simulink model "JX_Kinect_multi_sync"  (Simulink 7.7)
settings: Solver=ode4  StartTime=0.0  StopTime=inf  FixedStep=sample_time  RelTol=1e-3
InitFcn:
  | sample_time=0.005;%0.004;%0.0025;%0.02;
  | DeltaT = 0.02;
  | g = 9.81;
  | H0 = g%0.3165;
  | Kl = 1;
  | 
  | Omega_r = 1.6;%for Horizontal reference
  | Zeta_r = 1; %for Horizontal reference
  | Omega = 1.8;%for Horizontal Control
  | Zeta = 0.5;    %for Horizontal Control
  | 
  | Omega_h_r = 2.5; %for vertical reference
  | Zeta_h_r = 0.8;  %for vertical reference
  | Omega_h = 2.7;    %for vertical control
  | Zeta_h = 0.8;         %for vertical control
  | PI=pi;
  | 
  | Mass = 1.15;
  | Acc_Max = 4;
  | Acc_Max_h = 4;
  | 
  | Max_RP = 60;
  | 
  | % for NN
  | n = 5;
  | r = 3;
  | n2 = 5;
  | NN_ST = 0.02;
  | 
  | GAMA_V = 6;
  | gama_V_e = 0.01;
  | 
  | GAMA_W = GAMA_V;
  | gama_W_e =0.01;
  | 
  | % deadzone
  | NN_Deadzone_Z = 0;
  | 
  | % inputs nomalizaton parameters
  | NN_Z_y_min = -3;
  | NN_Z_y_max = 0.5;
  | 
  | NN_Z_v_max = 8;
  | NN_Z_v_min = -NN_Z_v_max;
  | 
  | % alpha = 0.034;
  | alpha = 1;
  | % c_f = 0.0015;
  | c_f = 0.001;
  | c_y_tilt = 1*0.5;
  | 
  | %for WK paras
  | Heightcontrol = 0.08;
  | Scale_Factor=1;
  | yoffset=0;
  | 
  | load MaoBi_Oct04_2_int.mat
  | MB_Interp.time = [];
undefined symbols (not defined in the file or in its folder): DiscIntNeverNeededParam
libraries: simulink x15, X330_Control x6, dspadpt3 x6, nid_lib x2
(part 4 of 4)

== system JX_Kinect_multi_sync/Vicon_Data/Raw Quad Pose from Vicon/Process Vicon Raw Data2/Flip_pi1/Flip_0_to_2pi/Flip_2pi ==
  Angle : Inport
  Bias : Bias  Bias=-2*pi
  Constant : Constant  Value=2*pi
  Data Type Duplicate : DataTypeDuplicate
  Modulo : Math  Operator=mod  SaturateOnIntegerOverflow=on
  Sign1 : Signum
  Switch : Switch
  Angle_Flip : Outport
  wires:
  Switch/1 -> Data Type Duplicate/2, Angle_Flip/1
  Bias/1 -> Switch/3
  Sign1/1 -> Switch/2
  Modulo/1 -> Switch/1, Bias/1
  Constant/1 -> Modulo/2
  Angle/1 -> Data Type Duplicate/1, Sign1/1, Modulo/1

== system JX_Kinect_multi_sync/Vicon_Data/Raw Quad Pose from Vicon/Process Vicon Raw Data3/Flip_pi1/Flip_0_to_2pi/Flip_2pi ==
  Angle : Inport
  Bias : Bias  Bias=-2*pi
  Constant : Constant  Value=2*pi
  Data Type Duplicate : DataTypeDuplicate
  Modulo : Math  Operator=mod  SaturateOnIntegerOverflow=on
  Sign1 : Signum
  Switch : Switch
  Angle_Flip : Outport
  wires:
  Angle/1 -> Modulo/1, Sign1/1, Data Type Duplicate/1
  Constant/1 -> Modulo/2
  Modulo/1 -> Bias/1, Switch/1
  Sign1/1 -> Switch/2
  Bias/1 -> Switch/3
  Switch/1 -> Angle_Flip/1, Data Type Duplicate/2

== system JX_Kinect_multi_sync/Vicon_Data/Raw Quad Pose from Vicon/Process Vicon Raw Data4/Flip_pi1/Flip_0_to_2pi/Flip_2pi ==
  Angle : Inport
  Bias : Bias  Bias=-2*pi
  Constant : Constant  Value=2*pi
  Data Type Duplicate : DataTypeDuplicate
  Modulo : Math  Operator=mod  SaturateOnIntegerOverflow=on
  Sign1 : Signum
  Switch : Switch
  Angle_Flip : Outport
  wires:
  Switch/1 -> Data Type Duplicate/2, Angle_Flip/1
  Bias/1 -> Switch/3
  Sign1/1 -> Switch/2
  Modulo/1 -> Switch/1, Bias/1
  Constant/1 -> Modulo/2
  Angle/1 -> Data Type Duplicate/1, Sign1/1, Modulo/1

== system JX_Kinect_multi_sync/Vicon_Data/Raw Quad Pose from Vicon/Process Vicon Raw Data6/Flip_pi1/Flip_0_to_2pi/Flip_2pi ==
  Angle : Inport
  Bias : Bias  Bias=-2*pi
  Constant : Constant  Value=2*pi
  Data Type Duplicate : DataTypeDuplicate
  Modulo : Math  Operator=mod  SaturateOnIntegerOverflow=on
  Sign1 : Signum
  Switch : Switch
  Angle_Flip : Outport
  wires:
  Angle/1 -> Modulo/1, Sign1/1, Data Type Duplicate/1
  Constant/1 -> Modulo/2
  Modulo/1 -> Bias/1, Switch/1
  Sign1/1 -> Switch/2
  Bias/1 -> Switch/3
  Switch/1 -> Angle_Flip/1, Data Type Duplicate/2

== system JX_Kinect_multi_sync/Vicon_Data/Raw Quad Pose from Vicon/Process Vicon Raw Data7/Flip_pi1/Flip_0_to_2pi/Flip_2pi ==
  Angle : Inport
  Bias : Bias  Bias=-2*pi
  Constant : Constant  Value=2*pi
  Data Type Duplicate : DataTypeDuplicate
  Modulo : Math  Operator=mod  SaturateOnIntegerOverflow=on
  Sign1 : Signum
  Switch : Switch
  Angle_Flip : Outport
  wires:
  Switch/1 -> Data Type Duplicate/2, Angle_Flip/1
  Bias/1 -> Switch/3
  Sign1/1 -> Switch/2
  Modulo/1 -> Switch/1, Bias/1
  Constant/1 -> Modulo/2
  Angle/1 -> Data Type Duplicate/1, Sign1/1, Modulo/1

== matlab function UAV1/Yaw Controller/MATLAB Function ==
  data: u input double; y output double
function y = fcn(u)
%#codegen
y = u;
if y > pi    
    y = y - 2*pi;
elseif y < -pi
        y = y + 2*pi;
end

== stateflow chart UAV2/Trajectory Logic/UAV SF ==
  state Landing
    state Descending
      en:PosDesired = Pos;
      du:PosDesired[2] = (0.1- PosDesired[2])*1*DeltaT + PosDesired[2] ;
    state CutThrottle
      en: PWM=1600;
      du:HoverThrottle = (0.0- HoverThrottle)*3*DeltaT + HoverThrottle ;
    (default) -> Descending
    Descending -> CutThrottle : [Pos[2] >(0.0 -0.1)]
  state AirBorne
    state TakeOff
      du:HoverThrottle = (H0 - HoverThrottle)*3*DeltaT + HoverThrottle ;
    state Kinect
      state Initialise
        en:
        PosDesired[0]=-1.5, PosDesired[1]=0,PosDesired[2]= -1.5,PosDesired[3]=0;
        LeftRight = 0;
        UpDown = 0;
        FrontBack = 0;
      state UpdateQuad
        en:
        PosDesired[0]=LeftRight, PosDesired[1]=FrontBack,PosDesired[2]=UpDown;
      state Kinect
        state FollowKinect
          en:
          LeftRight = KPos[3], FrontBack = KPos[4], UpDown = KPos[5];
          LH=1;
        state BoundaryContact
          en:
          LH=1;
        (default) -> (junction 41)
        (junction 41) -> BoundaryContact [order 2] : [((TooClose[0]==1)&(TooClose[2]==0))|((TooClose[0]==0)&(TooClose[2]==1))|(TooClose[3]==1)]
        (junction 41) -> FollowKinect [order 1] : [(TooClose[0]==0)&(TooClose[2]==0)]
      state Constraint
        state ALLGreen
          en:
          LH = 2;
        state PositionConstraint
          state Znegative
            en:
            UpDown=-2.5;
          state Ynegative
            en:
            FrontBack=-2;
          state Zpositive
            en:
            UpDown=-0.8;
          state Contained
            en:
            LH = 2;
          state Xpositive
            en:
            LeftRight=2;
          state Xnegative
            en:
            LeftRight=-2;
          state Ypositive
            en:
            FrontBack=2;
          Znegative -> Contained
          (junction 39) -> Zpositive [order 2] : [UpDown>-0.8]
          (junction 40) -> (junction 39) [order 1] : [FrontBack>=-2]
          Zpositive -> (junction 38)
          (junction 38) -> Znegative [order 2] : [UpDown<-2.5]
          (junction 39) -> (junction 38) [order 1] : [UpDown<=-0.8]
          (junction 38) -> Contained [order 1] : [UpDown>=-2.5]
          Ynegative -> (junction 39)
          (default) -> (junction 43)
          (junction 43) -> Xpositive [order 2] : [LeftRight>2]
          (junction 43) -> (junction 37) [order 1] : [LeftRight<=2]
          Xpositive -> (junction 37)
          (junction 37) -> Xnegative [order 2] : [LeftRight<-2]
          Xnegative -> (junction 36)
          (junction 37) -> (junction 36) [order 1] : [LeftRight>=-2]
          (junction 36) -> Ypositive [order 2] : [FrontBack>2]
          Ypositive -> (junction 40)
          (junction 36) -> (junction 40) [order 1] : [FrontBack<=2]
          (junction 40) -> Ynegative [order 2] : [FrontBack<-2]
        (default) -> (junction 42)
        (junction 42) -> ALLGreen [order 1] : [(LeftRight<=2)&(LeftRight>=-2)&(FrontBack<=2)&(FrontBack>=-2)&(UpDown<=-0.8)&(UpDown>=-2.5)]
        (junction 42) -> PositionConstraint [order 2] : [(LeftRight > 2)|(LeftRight<-2)|(FrontBack>2)|(FrontBack<-2)|(UpDown>-0.8)|(UpDown<-2.5)]
        PositionConstraint -> ALLGreen : [(LeftRight<=2)&(LeftRight>=-2)&(FrontBack<=2)&(FrontBack>=-2)&(UpDown<=-0.8)&(UpDown>=-2.5)]
      (default) -> Initialise
      Initialise -> UpdateQuad : after (3,sec)
      AirBorne.Kinect.Kinect -> UpdateQuad [order 1] : [KinectTracking==0]
      UpdateQuad -> AirBorne.Kinect.Kinect : [KinectTracking==1]
      Constraint -> UpdateQuad : [LH==2]
      AirBorne.Kinect.Kinect -> Constraint [order 2] : [LH==1]
    state Safety
      state Descent1
        descentrate=descentrate+0.02;
      state Prelanding
        en:PosDesired[0] = PerchPos[0]; PosDesired[1] = PerchPos[1];PosDesired[2] = PerchPos[2]-0.8 ;
        descentrate=0;
      state SafyHover
        en:PosDesired = Pos; PosDesired[2]= -1.5;
      state Descent
        en:PosDesired[0] = PerchPos[0]; PosDesired[1] = PerchPos[1];PosDesired[2] = PerchPos[2]-0.50+descentrate;
      Prelanding -> Descent : [PerchError < 0.01]
      Descent -> Descent1 [order 2] : [PerchError < 0.02]
      (default) -> SafyHover
      Descent -> Prelanding [order 1] : after (5,sec)
      Descent1 -> Descent : after (0.5,sec)
      SafyHover -> Prelanding : after (3, sec)
    (default) -> TakeOff : {PosDesired = Pos;  PosDesired[2] =-1.2;}
    TakeOff -> Safety [order 2] : [RC[5] > 0.5]
    TakeOff -> AirBorne.Kinect [order 1] : after (7,sec)
    AirBorne.Kinect -> Safety : [RC[5] > 0.5]
  (default) -> Landing : {HoverThrottle = 0;}
  AirBorne -> Landing : [RC[6] < -0.5]
  Landing -> AirBorne : [RC[6] > 0.5]
  data: PosDesired output double size=4; HoverThrottle output double size=1; Mode output uint8 size=1; RC input double size=8; Pos input double size=4; PerchPos input double size=4; DeltaT parameter double size=1; H0 parameter double size=1; Kl parameter double size=1; VelCmd local double size=2 =0; PWM output double; PerchError input double; KinectTracking input double; PI parameter double size=1; descentrate local double; KPos input double; UpDown local double; FrontBack local double; TooClose input double; LeftRight local double; XDiff local double; YDiff local double; diff local double; LH local double

== stateflow chart UAV1/Trajectory Logic/UAV SF ==
  state Landing
    state Descending
      en:PosDesired = Pos;
      du:PosDesired[2] = (0.1- PosDesired[2])*1*DeltaT + PosDesired[2] ;
    state CutThrottle
      en: PWM=1600;
      du:HoverThrottle = (0.0- HoverThrottle)*3*DeltaT + HoverThrottle ;
    (default) -> Descending
    Descending -> CutThrottle : [Pos[2] >(0.0 -0.1)]
  state AirBorne
    state TakeOff
      du:HoverThrottle = (H0 - HoverThrottle)*3*DeltaT + HoverThrottle ;
    state Kinect
      state Initialise
        en:
        PosDesired[0]=-1.5, PosDesired[1]=0,PosDesired[2]= -1.5,PosDesired[3]=0;
        LeftRight = 0;
        UpDown = 0;
        FrontBack = 0;
      state UpdateQuad
        en:
        PosDesired[0]=Pos2[0]+LeftRight, PosDesired[1]=Pos2[1]+FrontBack,PosDesired[2]= Pos2[2]+UpDown;
      state Kinect
        state FollowKinect
          en:
          LeftRight = KPos[0], FrontBack = KPos[1], UpDown = KPos[2];
          LH=1;
        state AtLeast2BoundaryContact
          state xright
            en:
            LeftRight = LeftRight+0.05;
            LH=1;
          state xleft
            en:
            LeftRight = LeftRight-0.05;
            LH=1;
          state yfront
            en:
            FrontBack = FrontBack-0.05;
            LH=1;
          state xright1
            en:
            FrontBack = FrontBack+0.05;
            LH=1;
          state quad3
            en:
            LH=1;
          (default) -> (junction 149)
          (junction 149) -> (junction 150) [order 2] : [TooClose[4]>TooClose[5]]
          (junction 149) -> (junction 151) [order 1] : [TooClose[5]>=TooClose[4]]
          (junction 150) -> (junction 152) [order 2] : [TooClose[6]==1]
          (junction 151) -> (junction 153) [order 1] : [TooClose[7]==1]
          (junction 152) -> xleft [order 2] : [KPos[0]<0]
          (junction 152) -> xright [order 1] : [KPos[0]>=0]
          (junction 153) -> yfront [order 2] : [KPos[1]<0]
          (junction 153) -> xright1 [order 1] : [KPos[1]>=0]
          (junction 150) -> quad3 [order 1] : [TooClose[6]==0]
          (junction 151) -> quad3 [order 2] : [TooClose[7]==0]
        state OneBoundaryContact
          en:
          LH=1;
        (default) -> (junction 154)
        (junction 154) -> AtLeast2BoundaryContact [order 2] : [TooClose[3]==1]
        (junction 154) -> FollowKinect [order 3] : [(TooClose[0]==0)&(TooClose[1]==0)]
        (junction 154) -> OneBoundaryContact [order 1] : [((TooClose[0]==1)&(TooClose[1]==0))|((TooClose[0]==10)&(TooClose[1]==1))]
      state Constraint
        state ALLGreen
          en:
          LH = 2;
        state PositionConstraint
          state Xpositive
            en:
            LeftRight=(2-Pos2[0]);
          state Xnegative
            en:
            LeftRight=(-2-Pos2[0]);
          state Ypositive
            en:
            FrontBack=(2-Pos2[1]);
          state Ynegative
            en:
            FrontBack=(-2-Pos2[1]);
          state Zpositive
            en:
            UpDown=(0.78-Pos2[2]);
          state Znegative
            en:
            UpDown=(-1-Pos2[2]);
          state Contained
            en:
            LH = 2;
          (default) -> (junction 156)
          (junction 156) -> Xpositive [order 2] : [LeftRight>(2-Pos2[0])]
          (junction 156) -> (junction 157) [order 1] : [LeftRight<=(2-Pos2[0])]
          Xpositive -> (junction 157)
          (junction 157) -> Xnegative [order 2] : [LeftRight<(-2-Pos2[0])]
          Xnegative -> (junction 158)
          (junction 157) -> (junction 158) [order 1] : [LeftRight>=(-2-Pos2[0])]
          (junction 158) -> Ypositive [order 2] : [FrontBack>(2-Pos2[1])]
          Ypositive -> (junction 159)
          (junction 158) -> (junction 159) [order 1] : [FrontBack<=(2-Pos2[1])]
          (junction 159) -> Ynegative [order 2] : [FrontBack<(-2-Pos2[1])]
          Ynegative -> (junction 160)
          (junction 159) -> (junction 160) [order 1] : [FrontBack>=(-2-Pos2[1])]
          (junction 160) -> Zpositive [order 2] : [UpDown>(0.78-Pos2[2])]
          Zpositive -> (junction 161)
          (junction 160) -> (junction 161) [order 1] : [UpDown<=(0.78-Pos2[2])]
          (junction 161) -> Znegative [order 2] : [UpDown<(-1-Pos2[2])]
          (junction 161) -> Contained [order 1] : [UpDown>=(-1-Pos2[2])]
          Znegative -> Contained
        (default) -> (junction 155)
        (junction 155) -> ALLGreen [order 1] : [(LeftRight<=(2-Pos2[0]))&(LeftRight>=(-2-Pos2[0]))&(FrontBack<=(2-Pos2[1]))&(FrontBack>=(-2-Pos2[1]))&(UpDown<=(0.78-Pos2[2]))&(UpDown>=(-1-Pos2[2]))]
        (junction 155) -> PositionConstraint [order 2] : [(LeftRight > (2-Pos2[0]))|(LeftRight<(-2-Pos2[0]))|(FrontBack>(2-Pos2[1]))|(FrontBack<(-2-Pos2[1]))|(UpDown>(0.78-Pos2[2]))|(UpDown<(-1-Pos2[2]))]
        PositionConstraint -> ALLGreen : [(LeftRight<=(2-Pos2[0]))&(LeftRight>=(-2-Pos2[0]))&(FrontBack<=(2-Pos2[1]))&(FrontBack>=(-2-Pos2[1]))&(UpDown<=(0.78-Pos2[2]))&(UpDown>=(-1-Pos2[2]))]
      (default) -> Initialise
      Initialise -> UpdateQuad : after (3,sec)
      AirBorne.Kinect.Kinect -> UpdateQuad [order 1] : [KinectTracking==0]
      UpdateQuad -> AirBorne.Kinect.Kinect : [KinectTracking==1]
      AirBorne.Kinect.Kinect -> Constraint [order 2] : [LH==1]
      Constraint -> UpdateQuad : [LH==2]
    state Safety
      state Descent1
        descentrate=descentrate+0.02;
      state Prelanding
        en:PosDesired[0] = PerchPos[0]; PosDesired[1] = PerchPos[1];PosDesired[2] = PerchPos[2]-0.8 ;
        descentrate=0;
      state SafyHover
        en:PosDesired = Pos; PosDesired[2]= -1.5;
      state Descent
        en:PosDesired[0] = PerchPos[0]; PosDesired[1] = PerchPos[1];PosDesired[2] = PerchPos[2]-0.50+descentrate;
      Prelanding -> Descent : [PerchError < 0.01]
      Descent -> Descent1 [order 2] : [PerchError < 0.02]
      (default) -> SafyHover
      Descent -> Prelanding [order 1] : after (5,sec)
      Descent1 -> Descent : after (0.5,sec)
      SafyHover -> Prelanding : after (3, sec)
    (default) -> TakeOff : {PosDesired = Pos;  PosDesired[2] =-1.2;}
    TakeOff -> Safety [order 2] : [RC[5] > 0.5]
    TakeOff -> AirBorne.Kinect [order 1] : after (7,sec)
    AirBorne.Kinect -> Safety : [RC[5] > 0.5]
  (default) -> Landing : {HoverThrottle = 0;}
  AirBorne -> Landing : [RC[6] < -0.5]
  Landing -> AirBorne : [RC[6] > 0.5]
  data: PosDesired output double size=4; HoverThrottle output double size=1; Mode output uint8 size=1; RC input double size=8; Pos input double size=4; PerchPos input double size=4; DeltaT parameter double size=1; H0 parameter double size=1; Kl parameter double size=1; VelCmd local double size=2 =0; PWM output double; PerchError input double; KinectTracking input double; PI parameter double size=1; descentrate local double; KPos input double; UpDown local double; FrontBack local double; TooClose input double; LeftRight local double; XDiff local double; YDiff local double; diff local double; LH local double; Pos2 input double

== matlab function UAV2/Yaw Controller/MATLAB Function ==
  data: u input double; y output double
function y = fcn(u)
%#codegen
y = u;
if y > pi    
    y = y - 2*pi;
elseif y < -pi
        y = y + 2*pi;
end

== matlab function Subsystem1/X Difference/MATLAB Function ==
  data: x1 input double; maxx output double; x2 input double; Quad output double
function [maxx,Quad] = xmax(x1,x2)

if (x1>x2)
    Quad = 1; 
    maxx = x1;             
else 
     Quad = 0;
     maxx = x2;          
end

end

== matlab function Subsystem1/Y Difference/MATLAB Function ==
  data: y1 input double; maxy output double; y2 input double; quady output double
function [maxy, quady]  = xmax(y1,y2)

if (y1>y2)
    quady = 1; %12 is the most
    maxy = y1;              
else 
     quady =0;
     maxy = y2;           
end

end

== matlab function Subsystem1/check if quad are too close ==
  data: Lx input double; Ly input double; Lz input double; Rx input double; Ry input double; Rz input double; Q1Q2 output double; Q1Q3 output double; Q2Q3 output double; TQ output double
function [Q1Q2, Q1Q3, Q2Q3, TQ] = quad_dist(Lx, Ly, Lz, Rx, Ry, Rz)

LQ2 = sqrt((Lx)^2 + (Ly)^2 + (Lz)^2);
LQ3 = sqrt((Lx-Rx)^2 + (Ly-Ry)^2 + (Lz-Rz)^2);

RQ2 = sqrt((Rx)^2 + (Ry)^2 + (Rz)^2);

if (LQ2 <= 1)
    Q1Q2 = 1;
else Q1Q2 = 0;
end

if (LQ3 <=1)
    Q1Q3 = 1;
else Q1Q3 =0;
end

if (RQ2 <=1)
    Q2Q3 = 1;
else Q2Q3 = 0;
end

if (((Q1Q2==1)&&(Q1Q3==1))||((Q1Q2==1)&&(Q2Q3==1))||((Q2Q3==1)&&(Q1Q2==1)))
    TQ=1;
end

end

== stateflow chart UAV3/Trajectory Logic/UAV SF ==
  state Landing
    state Descending
      en:PosDesired = Pos;
      du:PosDesired[2] = (0.1- PosDesired[2])*1*DeltaT + PosDesired[2] ;
    state CutThrottle
      en: PWM=1600;
      du:HoverThrottle = (0.0- HoverThrottle)*3*DeltaT + HoverThrottle ;
    (default) -> Descending
    Descending -> CutThrottle : [Pos[2] >(0.0 -0.1)]
  state AirBorne
    state TakeOff
      du:HoverThrottle = (H0 - HoverThrottle)*3*DeltaT + HoverThrottle ;
    state Kinect
      state Initialise
        en:
        PosDesired[0]=-1.5, PosDesired[1]=0,PosDesired[2]= -1.5,PosDesired[3]=0;
        LeftRight = 0;
        UpDown = 0;
        FrontBack = 0;
      state UpdateQuad
        en:
        PosDesired[0]=Pos2[0]+LeftRight, PosDesired[1]=Pos[2]+FrontBack,PosDesired[2]= Pos[2]+UpDown;
      state Kinect
        state FollowKinect
          en:
          LeftRight = KPos[6], FrontBack = KPos[7], UpDown = KPos[8];
          LH=1;
        state AtLeast2BoundaryContact
          state xright
            en:
            LeftRight = LeftRight+0.05;
            LH=1;
          state xleft
            en:
            LeftRight = LeftRight-0.05;
            LH=1;
          state yfront
            en:
            FrontBack = FrontBack-0.05;
            LH=1;
          state xright1
            en:
            FrontBack = FrontBack+0.05;
            LH=1;
          state quad1
            en:
            LH=1;
          (default) -> (junction 320)
          (junction 320) -> (junction 321) [order 2] : [TooClose[4]>TooClose[5]]
          (junction 320) -> (junction 322) [order 1] : [TooClose[5]>=TooClose[4]]
          (junction 321) -> (junction 323) [order 2] : [TooClose[6]==0]
          (junction 322) -> (junction 324) [order 1] : [TooClose[7]==0]
          (junction 323) -> xleft [order 2] : [KPos[6]<0]
          (junction 323) -> xright [order 1] : [KPos[6]>=0]
          (junction 324) -> yfront [order 2] : [KPos[7]<0]
          (junction 324) -> xright1 [order 1] : [KPos[7]>=0]
          (junction 322) -> quad1 [order 2] : [TooClose[7]==1]
          (junction 321) -> quad1 [order 1] : [TooClose[6]==1]
        state OneBoundaryContact
          en:
          LH=1;
        (default) -> (junction 325)
        (junction 325) -> AtLeast2BoundaryContact [order 2] : [TooClose[3]==1]
        (junction 325) -> FollowKinect [order 3] : [(TooClose[1]==0)&(TooClose[2]==0)]
        (junction 325) -> OneBoundaryContact [order 1] : [((TooClose[1]==1)&(TooClose[2]==0))|((TooClose[1]==0)&(TooClose[2]==1))]
      state Constraint
        state ALLGreen
          en:
          LH = 2;
        state PositionConstraint
          state Xpositive
            en:
            LeftRight=(2-Pos2[0]);
          state Xnegative
            en:
            LeftRight=(-2-Pos2[0]);
          state Ypositive
            en:
            FrontBack=(2-Pos2[1]);
          state Ynegative
            en:
            FrontBack=(-2-Pos2[1]);
          state Zpositive
            en:
            UpDown=(-0.8-Pos2[2]);
          state Znegative
            en:
            UpDown=(-2.5-Pos2[2]);
          state Contained
            en:
            LH = 2;
          (default) -> (junction 327)
          (junction 327) -> Xpositive [order 2] : [LeftRight>(2-Pos2[0])]
          (junction 327) -> (junction 328) [order 1] : [LeftRight<=(2-Pos2[0])]
          Xpositive -> (junction 328)
          (junction 328) -> Xnegative [order 2] : [LeftRight<(-2-Pos2[0])]
          Xnegative -> (junction 329)
          (junction 328) -> (junction 329) [order 1] : [LeftRight>=(-2-Pos2[0])]
          (junction 329) -> Ypositive [order 2] : [FrontBack>(2-Pos2[1])]
          Ypositive -> (junction 330)
          (junction 329) -> (junction 330) [order 1] : [FrontBack<=(2-Pos2[1])]
          (junction 330) -> Ynegative [order 2] : [FrontBack<(-2-Pos2[1])]
          Ynegative -> (junction 331)
          (junction 330) -> (junction 331) [order 1] : [FrontBack>=(-2-Pos2[1])]
          (junction 331) -> Zpositive [order 2] : [UpDown>(-0.8-Pos2[2])]
          Zpositive -> (junction 332)
          (junction 331) -> (junction 332) [order 1] : [UpDown<=(-0.8-Pos2[2])]
          (junction 332) -> Znegative [order 2] : [UpDown<(-2.5-Pos2[2])]
          (junction 332) -> Contained [order 1] : [UpDown>=(-2.5-Pos2[2])]
          Znegative -> Contained
        (default) -> (junction 326)
        (junction 326) -> ALLGreen [order 1] : [(LeftRight<=(2-Pos2[0]))&(LeftRight>=(-2-Pos2[0]))&(FrontBack<=(2-Pos2[1]))&(FrontBack>=(-2-Pos2[1]))&(UpDown<=(-0.8-Pos2[2]))&(UpDown>=(-2.5-Pos2[2]))]
        (junction 326) -> PositionConstraint [order 2] : [(LeftRight > 2)|(LeftRight<-2)|(FrontBack>2)|(FrontBack<-2)|(UpDown>0.78)|(UpDown<-1)]
        PositionConstraint -> ALLGreen : [(LeftRight<=(2-Pos2[0]))&(LeftRight>=(-2-Pos2[0]))&(FrontBack<=(2-Pos2[1]))&(FrontBack>=(-2-Pos2[1]))&(UpDown<=(-0.8-Pos2[2]))&(UpDown>=(-2.5-Pos2[2]))]
      (default) -> Initialise
      Initialise -> UpdateQuad : after (3,sec)
      AirBorne.Kinect.Kinect -> UpdateQuad [order 1] : [KinectTracking==0]
      UpdateQuad -> AirBorne.Kinect.Kinect : [KinectTracking==1]
      AirBorne.Kinect.Kinect -> Constraint [order 2] : [LH==1]
      Constraint -> UpdateQuad : [LH==2]
    state Safety
      state Descent1
        descentrate=descentrate+0.02;
      state Prelanding
        en:PosDesired[0] = PerchPos[0]; PosDesired[1] = PerchPos[1];PosDesired[2] = PerchPos[2]-0.8 ;
        descentrate=0;
      state SafyHover
        en:PosDesired = Pos; PosDesired[2]= -1.5;
      state Descent
        en:PosDesired[0] = PerchPos[0]; PosDesired[1] = PerchPos[1];PosDesired[2] = PerchPos[2]-0.50+descentrate;
      Prelanding -> Descent : [PerchError < 0.01]
      Descent -> Descent1 [order 2] : [PerchError < 0.02]
      (default) -> SafyHover
      Descent -> Prelanding [order 1] : after (5,sec)
      Descent1 -> Descent : after (0.5,sec)
      SafyHover -> Prelanding : after (3, sec)
    (default) -> TakeOff : {PosDesired = Pos;  PosDesired[2] =-1.2;}
    TakeOff -> Safety [order 2] : [RC[5] > 0.5]
    TakeOff -> AirBorne.Kinect [order 1] : after (7,sec)
    AirBorne.Kinect -> Safety : [RC[5] > 0.5]
  (default) -> Landing : {HoverThrottle = 0;}
  AirBorne -> Landing : [RC[6] < -0.5]
  Landing -> AirBorne : [RC[6] > 0.5]
  data: PosDesired output double size=4; HoverThrottle output double size=1; Mode output uint8 size=1; RC input double size=8; Pos input double size=4; PerchPos input double size=4; DeltaT parameter double size=1; H0 parameter double size=1; Kl parameter double size=1; VelCmd local double size=2 =0; PWM output double; PerchError input double; KinectTracking input double; PI parameter double size=1; descentrate local double; KPos input double; UpDown local double; FrontBack local double; TooClose input double; LeftRight local double; XDiff local double; YDiff local double; diff local double; LH local double; Pos2 input double

== matlab function UAV3/Yaw Controller/MATLAB Function ==
  data: u input double; y output double
function y = fcn(u)
%#codegen
y = u;
if y > pi    
    y = y - 2*pi;
elseif y < -pi
        y = y + 2*pi;
end
